simulink model "vst_ut"  (Simulink 8.1)
settings: Solver=FixedStepDiscrete  StartTime=0.0  StopTime=Inf  FixedStep=0.005  RelTol=1e-3
libraries: siltestlib x15, vst x1
settings Model: Creator=xsellart  LastModifiedBy=AT015555
settings DataIOCC: SignalLoggingSaveFormat=Dataset
settings OptimizationCC: ExpressionDepthLimit=128
settings DebuggingCC: FcnCallInpInsideContextMsg=EnableAllAsError
settings GRTTargetCC: CombineOutputUpdateFcns=on  GRTInterface=off

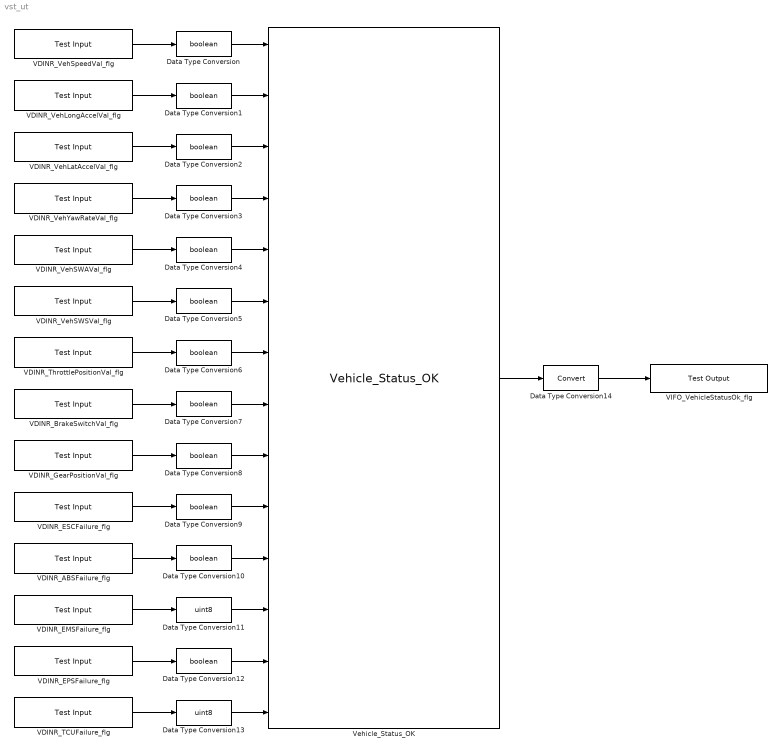
== system vst_ut ==
  Data Type Conversion{,1..10,12} (12 alike) : DataTypeConversion  OutDataTypeStr=boolean
  Data Type Conversion11 : DataTypeConversion  OutDataTypeStr=uint8
  Data Type Conversion13 : DataTypeConversion  OutDataTypeStr=uint8
  Data Type Conversion14 : DataTypeConversion
  "VDINR_ABSFailure_flg " : siltestlib/Test Input  varname=VDINR_ABSFault_flg  sampletime=0.005
  "VDINR_BrakeSwitchVal_flg " : siltestlib/Test Input  varname=VDINR_DriverBrakPedalOnValid_flg  sampletime=0.005
  "VDINR_EMSFailure_flg " : siltestlib/Test Input  varname=VDINR_EMSOpState_enum  sampletime=0.005
  "VDINR_EPSFailure_flg " : siltestlib/Test Input  varname=VDINR_EPASMILReq_flg  sampletime=0.005
  "VDINR_ESCFailure_flg " : siltestlib/Test Input  varname=VDINR_ESCFault_flg  sampletime=0.005
  "VDINR_GearPositionVal_flg " : siltestlib/Test Input  varname=VDINR_NowGearPosnValid_flg  sampletime=0.005
  "VDINR_TCUFailure_flg " : siltestlib/Test Input  varname=VDINR_TCMFaultStatus_enum  sampletime=0.005
  "VDINR_ThrottlePositionVal_flg " : siltestlib/Test Input  varname=VDINR_HWAccelPedalPosnValid_flg  sampletime=0.005
  "VDINR_VehLatAccelVal_flg " : siltestlib/Test Input  varname=VDINR_LatAccelValid_flg  sampletime=0.005
  "VDINR_VehLongAccelVal_flg " : siltestlib/Test Input  varname=VDINR_LongAccelValid_flg  sampletime=0.005
  "VDINR_VehSWAVal_flg " : siltestlib/Test Input  varname=VDINR_SteerAngleValid_flg  sampletime=0.005
  "VDINR_VehSWSVal_flg " : siltestlib/Test Input  varname=VDINR_SteerSpeedValid_flg  sampletime=0.005
  "VDINR_VehSpeedVal_flg " : siltestlib/Test Input  varname=VDINR_VehSpdValid_flg  sampletime=0.005
  "VDINR_VehYawRateVal_flg " : siltestlib/Test Input  varname=VDINR_YawRateValid_flg  sampletime=0.005
  "VIFO_VehicleStatusOk_flg " : siltestlib/Test Output  varname=VIFO_VehicleStatusOk_flg  sampletime=-1
  Vehicle_Status_OK : vst/Vehicle_Status_OK
  wires:
  "VDINR_VehSpeedVal_flg "/1 -> Data Type Conversion/1
  Data Type Conversion/1 -> Vehicle_Status_OK/1
  Vehicle_Status_OK/1 -> Data Type Conversion14/1
  Data Type Conversion14/1 -> "VIFO_VehicleStatusOk_flg "/1
  "VDINR_VehLongAccelVal_flg "/1 -> Data Type Conversion1/1
  Data Type Conversion1/1 -> Vehicle_Status_OK/2
  "VDINR_VehLatAccelVal_flg "/1 -> Data Type Conversion2/1
  Data Type Conversion2/1 -> Vehicle_Status_OK/3
  "VDINR_VehYawRateVal_flg "/1 -> Data Type Conversion3/1
  Data Type Conversion3/1 -> Vehicle_Status_OK/4
  "VDINR_VehSWAVal_flg "/1 -> Data Type Conversion4/1
  Data Type Conversion4/1 -> Vehicle_Status_OK/5
  "VDINR_VehSWSVal_flg "/1 -> Data Type Conversion5/1
  Data Type Conversion5/1 -> Vehicle_Status_OK/6
  "VDINR_ThrottlePositionVal_flg "/1 -> Data Type Conversion6/1
  Data Type Conversion6/1 -> Vehicle_Status_OK/7
  "VDINR_BrakeSwitchVal_flg "/1 -> Data Type Conversion7/1
  Data Type Conversion7/1 -> Vehicle_Status_OK/8
  "VDINR_GearPositionVal_flg "/1 -> Data Type Conversion8/1
  Data Type Conversion8/1 -> Vehicle_Status_OK/9
  "VDINR_ESCFailure_flg "/1 -> Data Type Conversion9/1
  Data Type Conversion9/1 -> Vehicle_Status_OK/10
  "VDINR_ABSFailure_flg "/1 -> Data Type Conversion10/1
  Data Type Conversion10/1 -> Vehicle_Status_OK/11
  "VDINR_EMSFailure_flg "/1 -> Data Type Conversion11/1
  Data Type Conversion11/1 -> Vehicle_Status_OK/12
  "VDINR_EPSFailure_flg "/1 -> Data Type Conversion12/1
  Data Type Conversion12/1 -> Vehicle_Status_OK/13
  "VDINR_TCUFailure_flg "/1 -> Data Type Conversion13/1
  Data Type Conversion13/1 -> Vehicle_Status_OK/14
